simulink model "bandwidth_force_sea"  (R2020b)
settings: Solver=ode4  StartTime=0.0  StopTime=10  FixedStep=1e-5  MaxStep=1e-4  RelTol=1e-4  EnableMultiTasking=on
values from neighbouring files (symbols this model uses):
  Be = 2 * sqrt(Ke * Je)    [bandwidth.m]    (also in bandwidth_reference.m = 2 * sqrt(Ke * 0.0001); frequency_max_modulation_force_sea.m = 0.2)
  D = 0.1    [bandwidth.m]    (also in bandwidth_reference.m = 0.9; frequency_max_modulation_force.m = 0.9; frequency_max_modulation_force_sea.m = 0.9; frequency_max_modulation_position.m = 0.9)
  dm = 0.0068    [bandwidth.m]    (also in bandwidth_reference.m; frequency_max_modulation_force.m; frequency_max_modulation_force_sea.m; frequency_max_modulation_position.m)
  FF = 0    [bandwidth.m]    (also in bandwidth_reference.m; frequency_max_modulation_force_sea.m; frequency_max_position.m; frequency_max_velocity.m)
  Je = 1e-1    (= 0.1)    [bandwidth.m]    (also in frequency_max_modulation_force_sea.m = 0)
  Jm = 0.0064    [bandwidth.m]    (also in bandwidth_reference.m = 0.0104; frequency_max_modulation_force.m = 0.0104; frequency_max_modulation_force_sea.m = 0.0104; frequency_max_modulation_position.m = 0.0104)
  Ke = 1e-2    (= 0.01)    [bandwidth.m]    (also in bandwidth_reference.m = 20; frequency_max_modulation_force_sea.m = 50)
  Ks = 12.04    [bandwidth.m]    (also in frequency_max_modulation_force_sea.m = 10)
  kt = 1.5038    [bandwidth_reference.m]    (also in frequency_max_modulation_force.m; frequency_max_modulation_force_sea.m; frequency_max_modulation_position.m; frequency_max_modulation_velocity.m)
  P = 15    [bandwidth.m]    (also in bandwidth_reference.m = 1; frequency_max_modulation_force.m = 10; frequency_max_modulation_force_sea.m = 10; frequency_max_modulation_position.m = 10)
settings Model: Creator=eldisondimo  LastModifiedBy=filippo
settings DataIOCC: LimitDataPoints=on  SaveOutput=off  SaveTime=off  ReturnWorkspaceOutputs=off
settings OptimizationCC: ExpressionDepthLimit=2147483647  LifeSpan=1
settings DebuggingCC: UnderspecifiedInitializationDetection=Classic  MergeDetectMultiDrivingBlocksExec=none  FcnCallInpInsideContextMsg=warning  AllowSymbolicDim=off  StateNameClashWarn=warning  SFUnexpectedBacktrackingDiag=warning  SFNoUnconditionalDefaultTransitionDiag=warning  SFExecutionAtInitializationDiag=none  ArithmeticOperatorsInVariantConditions=warning
settings SFSimCC: SimUseLocalCustomCode=off  CustomCodeUndefinedFunction=UseInterfaceOnly
settings RTWCC: RTWUseLocalCustomCode=off
settings CodeAppCC: StateflowObjectComments=on
settings GRTTargetCC: TargetLangStandard=C89/C90 (ANSI)  CombineOutputUpdateFcns=off  GRTInterface=on

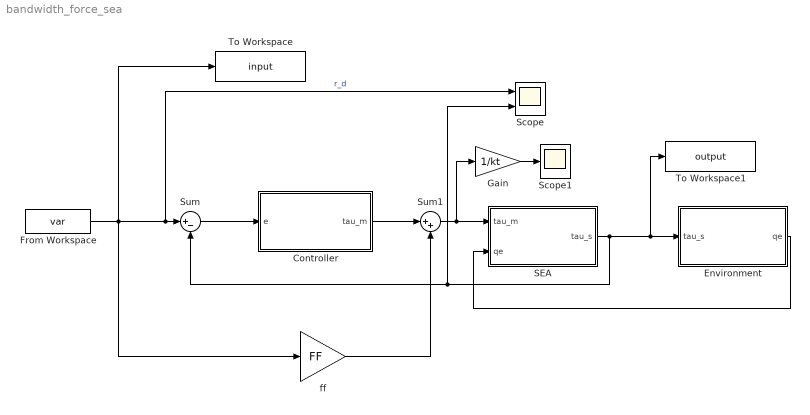
== system bandwidth_force_sea ==
  Controller : Subsystem
  Environment : Subsystem
  From Workspace : FromWorkspace  VariableName=var
  Gain : Gain  Gain=1/kt
  SEA : Subsystem
  Scope : Scope  NumInputPorts=2
  Scope1 : Scope
  Sum : Sum  Inputs=|+-
  Sum1 : Sum  Inputs=|++
  To Workspace : ToWorkspace  VariableName=input  SaveFormat=Structure With Time  SampleTime=-1
  To Workspace1 : ToWorkspace  VariableName=output  SaveFormat=Structure With Time  SampleTime=-1
  "ff " : Gain  Gain=FF
  wires:
  Sum/1 -> Controller/1(e)
  SEA/1(tau_s) -> To Workspace1/1, Environment/1(tau_s), Scope/2, Sum/2
  Controller/1(tau_m) -> Sum1/1
  Environment/1(qe) -> SEA/2("qe ")
  "ff "/1 -> Sum1/2
  From Workspace/1 -> "ff "/1, To Workspace/1, Scope/1, Sum/1  "r_d"
  Sum1/1 -> Gain/1, SEA/1(tau_m)
  Gain/1 -> Scope1/1

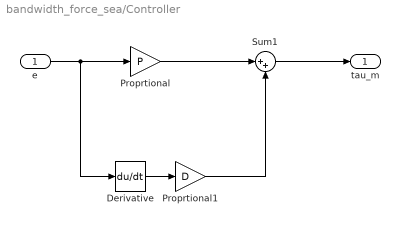
== system bandwidth_force_sea/Controller ==
  e : Inport
  Derivative : Derivative
  Proprtional : Gain  Gain=P
  Proprtional1 : Gain  Gain=D
  Sum1 : Sum  Inputs=|++
  tau_m : Outport  VectorParamsAs1DForOutWhenUnconnected=off
  wires:
  e/1 -> Derivative/1, Proprtional/1
  Sum1/1 -> tau_m/1
  Derivative/1 -> Proprtional1/1
  Proprtional/1 -> Sum1/1
  Proprtional1/1 -> Sum1/2

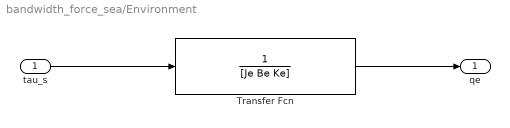
== system bandwidth_force_sea/Environment ==
  tau_s : Inport
  Transfer Fcn : TransferFcn  Denominator=[Je Be Ke]
  qe : Outport  VectorParamsAs1DForOutWhenUnconnected=off
  wires:
  tau_s/1 -> Transfer Fcn/1
  Transfer Fcn/1 -> qe/1

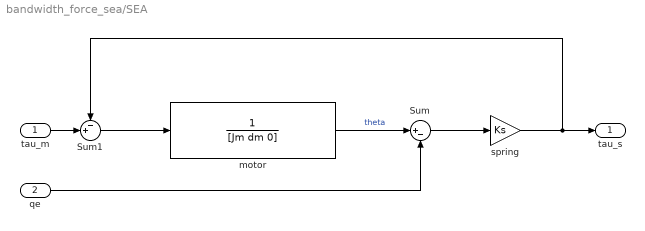
== system bandwidth_force_sea/SEA ==
  tau_m : Inport
  "qe " : Inport  Port=2
  Sum : Sum  Inputs=|+-
  Sum1 : Sum  Inputs=-+|
  "motor " : TransferFcn  Denominator=[Jm dm 0]
  "spring " : Gain  Gain=Ks
  tau_s : Outport  VectorParamsAs1DForOutWhenUnconnected=off
  wires:
  "motor "/1 -> Sum/1  "theta"
  "qe "/1 -> Sum/2
  Sum/1 -> "spring "/1
  "spring "/1 -> Sum1/1, tau_s/1
  tau_m/1 -> Sum1/2
  Sum1/1 -> "motor "/1
